simulink model "LQ"  (R2020b)
settings: Solver=ode1be  StartTime=0.0  StopTime=10  FixedStep=0.01  RelTol=1e-3
undefined symbols (not defined in the file or in its folder): Lr, Ly
settings Model: ODK_VersionTypeOld=V2.5  Creator=Mehrab  LastModifiedBy=Mehrab
settings DataIOCC: LimitDataPoints=on  SaveFormat=Array  SaveOutput=off  SaveTime=off
settings OptimizationCC: LifeSpan=1
settings DebuggingCC: FrameProcessingCompatibilityMsg=none
settings HardwareCC: ProdBitPerPointer=32  ProdBitPerSizeT=32  ProdBitPerPtrDiffT=32  ProdWordSize=32  ProdHWDeviceType=Intel->x86-32 (Windows32)
settings RTWCC: Description=Target for ODK capable S7-1500 Controllers based on Simulink Coder  SystemTargetFile=Target_1500S_V4_0_grt.tlc  TLCOptions=-aAlwaysIncludeCustomSrc=1  GenCodeOnly=on  GenerateMakefile=off  TemplateMakefile=Target_1500S_V4_0_grt.tmf  RTWVerbose=off  TargetLang=C++
settings CodeAppCC: MaxIdLength=256
settings STFCustomTargetCC: TargetLangStandard=C++03 (ISO)  ParMdlRefBuildCompliant=on  ConcurrentExecutionCompliant=off  CombineOutputUpdateFcns=on  CPPClassGenCompliant=off  GRTInterface=off  SystemTargetFile=Target_1500S_V4_0_grt.tlc
settings GRTTargetCC: TargetLangStandard=C++03 (ISO)  CompOptLevelCompliant=off  ConcurrentExecutionCompliant=off  MatFileLogging=off  CPPClassGenCompliant=off  UseToolchainInfoCompliant=off  ExtModeStaticAlloc=on  ExtModeMexFile=mwsl_ii_ext_comm_target1500s_v4  ExtModeMexArgs='192.168.3.3' 0 17725 0

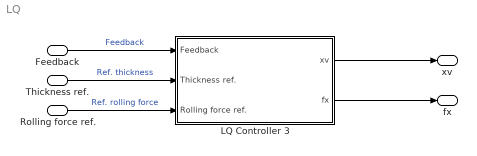
== system LQ ==
  Feedback : Inport  OutDataTypeStr=double  PortDimensions=5  SampleTime=[0.01 0]  Interpolate=off
  Thickness ref. : Inport  Port=2  OutDataTypeStr=double  PortDimensions=1  SampleTime=[-1 0]  Interpolate=off
  Rolling force ref. : Inport  Port=3  OutDataTypeStr=double  PortDimensions=1  SampleTime=[-1 0]  Interpolate=off
  LQ Controller 3 : Subsystem  Tag=RollingMill_SIM_Discrete
  xv : Outport  OutDataTypeStr=double  PortDimensions=1  SampleTime=[0.01 0]
  fx : Outport  Port=2  OutDataTypeStr=double  PortDimensions=1  SampleTime=[0.01 0]
  wires:
  Feedback/1 -> LQ Controller 3/1(Feedback)  "Feedback"
  Thickness ref./1 -> LQ Controller 3/2(Thickness ref.)  "Ref. thickness"
  Rolling force ref./1 -> LQ Controller 3/3(Rolling force ref.)  "Ref. rolling force"
  LQ Controller 3/1(xv) -> xv/1
  LQ Controller 3/2(fx) -> fx/1

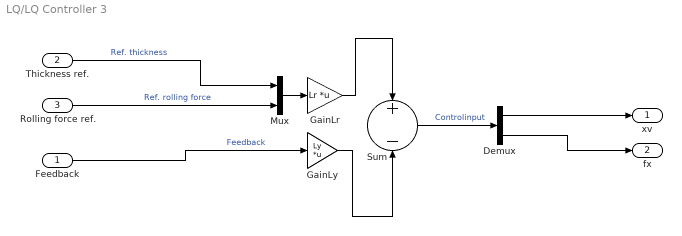
== system LQ/LQ Controller 3 ==
  Feedback : Inport
  Thickness ref. : Inport  Port=2
  Rolling force ref. : Inport  Port=3
  Demux : Demux  Outputs=2
  GainLr : Gain  Gain=Lr  Multiplication=Matrix(K*u)
  GainLy : Gain  Gain=Ly  Multiplication=Matrix(K*u)
  Mux : Mux  Inputs=2
  Sum : Sum  Inputs=+-
  xv : Outport
  fx : Outport  Port=2
  wires:
  Demux/2 -> fx/1
  Demux/1 -> xv/1
  GainLr/1 -> Sum/1
  Mux/1 -> GainLr/1
  Rolling force ref./1 -> Mux/2  "Ref. rolling force"
  Feedback/1 -> GainLy/1  "Feedback"
  Thickness ref./1 -> Mux/1  "Ref. thickness"
  GainLy/1 -> Sum/2
  Sum/1 -> Demux/1  "Controlinput"
